simulink model "sampleModel1588"  (R2023a)
settings: Solver=VariableStepAuto  StartTime=0.0  StopTime=10.0  RelTol=1e-3
libraries: hdlsllib x9
settings Model: Creator=user1  LastModifiedBy=user1

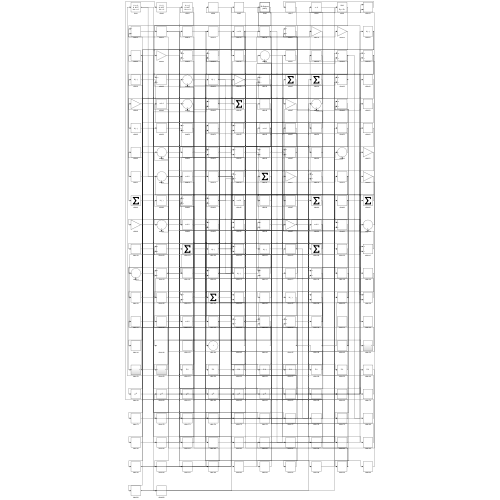
[thumbnail: Simulink's stored preview of the top-level diagram]
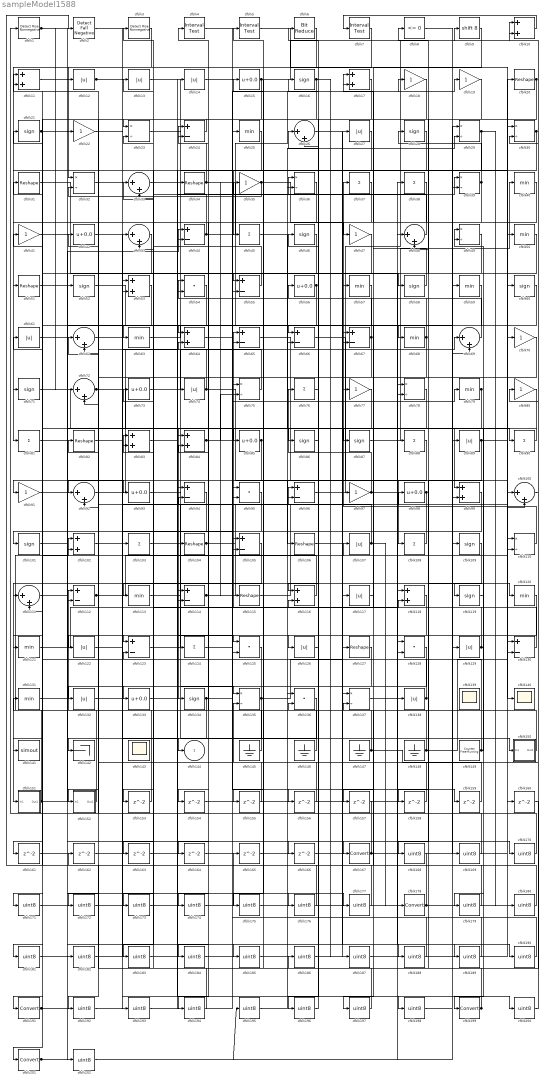
== system sampleModel1588 ==
  cfblk1 : hdlsllib/Logic and Bit Operations/Detect Rise Nonnegative  vinit=0  OutDataTypeStr=boolean
  cfblk{10..11,17,53,64,83..84,99,102,116,118} (11 alike) : Sum
  cfblk{26,33,43,48,62,69,72,92,100,111} (10 alike) : Sum  Inputs=|++
  cfblk{16,21,28,46,52,58,60,71,86..87,101,109,119,134} (14 alike) : Signum
  cfblk{37..38,45,76,81,88,90,103,108,124} (10 alike) : Sum  Inputs=+
  cfblk{20,31,34,51,82,104,106,115,127} (9 alike) : Reshape
  cfblk{24,44,55,65..67,94,96,105,112,114,123,130} (13 alike) : Sum  Inputs=+-
  cfblk{12..14,27,61,74,89,107,117,122,126,129,132,138} (14 alike) : Abs  SaturateOnIntegerOverflow=off
  cfblk{23,29..30,32,36,39,49,75,78,110,135,137} (12 alike) : Product  Inputs=*/  RndMeth=Zero  SaturateOnIntegerOverflow=on
  cfblk{25,40,50,57,59,63,68,79,113,120..121,131} (12 alike) : MinMax
  cfblk{54,95,125,128,136} (5 alike) : DotProduct  OutDataTypeStr=Inherit: Inherit via internal rule
  cfblk{15,42,56,73,85,93,98,133} (8 alike) : Bias  Bias=0.0  SaturateOnIntegerOverflow=off
  cfblk139 : Scope
      settings: Floating=on
  cfblk140 : Scope
  cfblk141 : ToWorkspace  VariableName=simout  SaveFormat=Timeseries  SampleTime=-1
  cfblk142 : Terminator
  cfblk143 : Scope
      settings: Floating=on
  cfblk{145..148} (4 alike) : Ground
  cfblk149 : hdlsllib/Sources/Counter Free-Running  NumBits=16  tsamp=-1
  cfblk150 : Subsystem
      settings: LibrarySourceBlock=|
      | hdlsllib/Ports &
      | Subsystems/Subsystem
  cfblk151 : Subsystem
      settings: LibrarySourceBlock=|
      | hdlsllib/Ports &
      | Subsystems/Subsystem
  cfblk152 : Subsystem
      settings: LibrarySourceBlock=|
      | hdlsllib/Ports &
      | Subsystems/Subsystem
  cfblk{153..166} (14 alike) : Delay  SampleTime=1
  cfblk{167,178,191,199,201} (5 alike) : DataTypeConversion  SaturateOnIntegerOverflow=off  RndMeth=Floor
  cfblk{168..177,179..190,192..198,200,202} (31 alike) : DataTypeConversion  OutDataTypeStr=uint8  SaturateOnIntegerOverflow=off  RndMeth=Floor
  cfblk{18..19,22,35,41,47,70,77,80,91,97} (11 alike) : Gain
  cfblk2 : hdlsllib/Logic and Bit Operations/Detect Fall Negative  vinit=0  OutDataTypeStr=boolean
  cfblk3 : hdlsllib/Logic and Bit Operations/Detect Rise Nonnegative  vinit=0  OutDataTypeStr=boolean
  cfblk4 : hdlsllib/Logic and Bit Operations/Interval Test  IntervalClosedRight=on  uplimit=0.5  IntervalClosedLeft=on  lowlimit=-0.5  OutDataTypeStr=boolean
  cfblk5 : hdlsllib/Logic and Bit Operations/Interval Test  IntervalClosedRight=on  uplimit=0.5  IntervalClosedLeft=on  lowlimit=-0.5  OutDataTypeStr=boolean
  cfblk6 : hdlsllib/Logic and Bit Operations/Bit Reduce  mode=AND
  cfblk7 : hdlsllib/Logic and Bit Operations/Interval Test  IntervalClosedRight=on  uplimit=0.5  IntervalClosedLeft=on  lowlimit=-0.5  OutDataTypeStr=boolean
  cfblk8 : hdlsllib/Logic and Bit Operations/Compare To Zero  relop=<=  OutDataTypeStr=boolean
  cfblk9 : ArithShift  BitShiftNumber=8
  cfblk144 : Outport  VectorParamsAs1DForOutWhenUnconnected=off
  wires:
  cfblk137/1 -> cfblk178/1
  cfblk7/1 -> cfblk32/1
  cfblk110/1 -> cfblk37/1
  cfblk1/1 -> cfblk72/1, cfblk170/1
  cfblk150/1(Out1) -> cfblk112/1
  cfblk121/1 -> cfblk65/1
  cfblk151/1(Out1) -> cfblk102/1, cfblk44/2
  cfblk29/1 -> cfblk123/1, cfblk72/2, cfblk180/1
  cfblk9/1 -> cfblk81/1
  cfblk46/1 -> cfblk125/1
  cfblk49/1 -> cfblk65/2
  cfblk28/1 -> cfblk112/2
  cfblk147/1 -> cfblk10/1, cfblk24/2
  cfblk13/1 -> cfblk150/1(In1)
  cfblk3/1 -> cfblk71/1
  cfblk105/1 -> cfblk151/1(In1)
  cfblk123/1 -> cfblk96/1
  cfblk95/1 -> cfblk191/1
  cfblk93/1 -> cfblk120/1
  cfblk73/1 -> cfblk69/1
  cfblk38/1 -> cfblk201/1
  cfblk18/1 -> cfblk47/1
  cfblk107/1 -> cfblk82/1, cfblk138/1
  cfblk116/1 -> cfblk11/1
  cfblk79/1 -> cfblk134/1, cfblk152/1(In1)
  cfblk54/1 -> cfblk132/1
  cfblk96/1 -> cfblk9/1
  cfblk118/1 -> cfblk122/1
  cfblk2/1 -> cfblk167/1
  cfblk65/1 -> cfblk108/1
  cfblk63/1 -> cfblk66/1
  cfblk122/1 -> cfblk97/1
  cfblk52/1 -> cfblk64/1
  cfblk66/1 -> cfblk140/1
  cfblk71/1 -> cfblk99/1
  cfblk106/1 -> cfblk67/1
  cfblk4/1 -> cfblk25/1
  cfblk97/1 -> cfblk76/1, cfblk190/1
  cfblk47/1 -> cfblk66/2
  cfblk148/1 -> cfblk110/1, cfblk35/1
  cfblk69/1 -> cfblk54/1
  cfblk132/1 -> cfblk103/1
  cfblk108/1 -> cfblk104/1
  cfblk85/1 -> cfblk94/1, cfblk161/1
  cfblk86/1 -> cfblk56/1
  cfblk44/1 -> cfblk19/1, cfblk23/2
  cfblk111/1 -> cfblk52/1
  cfblk89/1 -> cfblk100/2, cfblk158/1
  cfblk129/1 -> cfblk17/1, cfblk49/1
  cfblk25/1 -> cfblk51/1
  cfblk113/1 -> cfblk135/1
  cfblk134/1 -> cfblk142/1, cfblk118/2
  cfblk40/1 -> cfblk114/1
  cfblk33/1 -> cfblk125/2
  cfblk39/1 -> cfblk28/1, cfblk101/1
  cfblk53/1 -> cfblk63/1
  cfblk90/1 -> cfblk86/1
  cfblk92/1 -> cfblk14/1
  cfblk6/1 -> cfblk12/1
  cfblk146/1 -> cfblk41/1
  cfblk112/1 -> cfblk60/1, cfblk119/1
  cfblk138/1 -> cfblk83/1, cfblk44/1
  cfblk32/1 -> cfblk144/1
  cfblk12/1 -> cfblk53/1, cfblk166/1
  cfblk80/1 -> cfblk199/1
  cfblk34/1 -> cfblk129/1, cfblk24/1, cfblk115/1
  cfblk55/1 -> cfblk3/1
  cfblk81/1 -> cfblk90/1
  cfblk72/1 -> cfblk109/1, cfblk64/2
  cfblk83/1 -> cfblk39/1
  cfblk99/1 -> cfblk141/1
  cfblk98/1 -> cfblk163/1, cfblk196/1
  cfblk10/1 -> cfblk7/1
  cfblk87/1 -> cfblk40/1
  cfblk67/1 -> cfblk46/1, cfblk92/2
  cfblk75/1 -> cfblk11/2
  cfblk16/1 -> cfblk85/1, cfblk187/1
  cfblk35/1 -> cfblk127/1, cfblk32/2
  cfblk58/1 -> cfblk17/2
  cfblk24/1 -> cfblk22/1
  cfblk20/1 -> cfblk58/1, cfblk126/1
  cfblk152/1(Out1) -> cfblk31/1
  cfblk125/1 -> cfblk123/2
  cfblk114/1 -> cfblk50/1, cfblk99/2, cfblk88/1
  cfblk68/1 -> cfblk36/1, cfblk173/1
  cfblk21/1 -> cfblk67/2, cfblk121/1
  cfblk57/1 -> cfblk124/1
  cfblk27/1 -> cfblk114/2
  cfblk84/1 -> cfblk75/2, cfblk156/1
  cfblk17/1 -> cfblk53/2
  cfblk145/1 -> cfblk21/1
  cfblk36/1 -> cfblk113/1
  cfblk104/1 -> cfblk29/1, cfblk79/1
  cfblk45/1 -> cfblk87/1
  cfblk128/1 -> cfblk133/1
  cfblk56/1 -> cfblk91/1, cfblk155/1
  cfblk149/1 -> cfblk84/2, cfblk49/2
  cfblk115/1 -> cfblk98/1
  cfblk130/1 -> cfblk83/2
  cfblk100/1 -> cfblk30/2
  cfblk37/1 -> cfblk92/1
  cfblk19/1 -> cfblk23/1
  cfblk74/1 -> cfblk128/2, cfblk33/2, cfblk106/1, cfblk130/2
  cfblk15/1 -> cfblk10/2, cfblk111/1, cfblk111/2, cfblk55/1
  cfblk102/1 -> cfblk94/2
  cfblk30/1 -> cfblk45/1, cfblk175/1
  cfblk76/1 -> cfblk116/1
  cfblk23/1 -> cfblk130/1
  cfblk117/1 -> cfblk57/1
  cfblk50/1 -> cfblk62/2
  cfblk135/1 -> cfblk61/1, cfblk117/1, cfblk29/2, cfblk172/1
  cfblk64/1 -> cfblk18/1
  cfblk11/1 -> cfblk93/1
  cfblk31/1 -> cfblk118/1
  cfblk51/1 -> cfblk68/1
  cfblk133/1 -> cfblk107/1
  cfblk48/1 -> cfblk4/1
  cfblk124/1 -> cfblk116/2
  cfblk82/1 -> cfblk105/2
  cfblk126/1 -> cfblk16/1
  cfblk5/1 -> cfblk110/2
  cfblk94/1 -> cfblk153/1
  cfblk153/1 -> cfblk102/2
  cfblk60/1 -> cfblk154/1
  cfblk154/1 -> cfblk48/1
  cfblk155/1 -> cfblk105/1
  cfblk156/1 -> cfblk135/2
  cfblk120/1 -> cfblk157/1
  cfblk157/1 -> cfblk1/1
  cfblk158/1 -> cfblk128/1
  cfblk14/1 -> cfblk159/1
  cfblk159/1 -> cfblk62/1
  cfblk161/1 -> cfblk54/2
  cfblk162/1 -> cfblk30/1
  cfblk88/1 -> cfblk164/1
  cfblk164/1 -> cfblk36/2
  cfblk165/1 -> cfblk100/1
  cfblk166/1 -> cfblk6/1
  cfblk167/1 -> cfblk20/1, cfblk42/1, cfblk5/1
  cfblk109/1 -> cfblk168/1
  cfblk168/1 -> cfblk2/1
  cfblk8/1 -> cfblk169/1
  cfblk169/1 -> cfblk73/1
  cfblk170/1 -> cfblk8/1
  cfblk78/1 -> cfblk171/1
  cfblk171/1 -> cfblk27/1
  cfblk172/1 -> cfblk78/1
  cfblk173/1 -> cfblk78/2
  cfblk70/1 -> cfblk174/1
  cfblk174/1 -> cfblk165/1
  cfblk175/1 -> cfblk70/1
  cfblk131/1 -> cfblk176/1
  cfblk176/1 -> cfblk84/1
  cfblk91/1 -> cfblk177/1
  cfblk177/1 -> cfblk131/1
  cfblk178/1 -> cfblk96/2, cfblk33/1
  cfblk119/1 -> cfblk179/1
  cfblk179/1 -> cfblk137/1
  cfblk180/1 -> cfblk137/2
  cfblk43/1 -> cfblk181/1
  cfblk181/1 -> cfblk74/1
  cfblk61/1 -> cfblk182/1
  cfblk182/1 -> cfblk43/1
  cfblk163/1 -> cfblk183/1
  cfblk183/1 -> cfblk43/2
  cfblk77/1 -> cfblk184/1
  cfblk184/1 -> cfblk89/1
  cfblk101/1 -> cfblk185/1
  cfblk185/1 -> cfblk77/1
  cfblk160/1 -> cfblk186/1
  cfblk186/1 -> cfblk39/2
  cfblk187/1 -> cfblk160/1
  cfblk26/1 -> cfblk188/1
  cfblk188/1 -> cfblk75/1
  cfblk42/1 -> cfblk189/1
  cfblk189/1 -> cfblk26/1
  cfblk190/1 -> cfblk26/2
  cfblk191/1 -> cfblk55/2, cfblk34/1
  cfblk127/1 -> cfblk192/1
  cfblk192/1 -> cfblk95/1
  cfblk62/1 -> cfblk193/1
  cfblk193/1 -> cfblk95/2
  cfblk136/1 -> cfblk194/1
  cfblk194/1 -> cfblk13/1
  cfblk195/1 -> cfblk136/1
  cfblk196/1 -> cfblk136/2
  cfblk59/1 -> cfblk197/1
  cfblk197/1 -> cfblk162/1
  cfblk22/1 -> cfblk198/1
  cfblk198/1 -> cfblk59/1
  cfblk199/1 -> cfblk48/2, cfblk15/1
  cfblk103/1 -> cfblk200/1
  cfblk200/1 -> cfblk80/1
  cfblk201/1 -> cfblk195/1, cfblk69/2
  cfblk41/1 -> cfblk202/1
  cfblk202/1 -> cfblk38/1

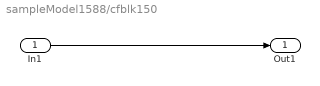
== system sampleModel1588/cfblk150 ==
  In1 : Inport
  Out1 : Outport
  wires:
  In1/1 -> Out1/1

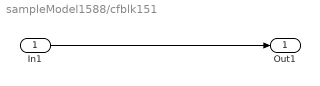
== system sampleModel1588/cfblk151 ==
  In1 : Inport
  Out1 : Outport
  wires:
  In1/1 -> Out1/1

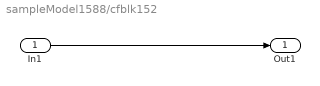
== system sampleModel1588/cfblk152 ==
  In1 : Inport
  Out1 : Outport
  wires:
  In1/1 -> Out1/1
